simulink library "My_FI_Operations"  (R2023a)
settings: Solver=VariableStepAuto  StartTime=0.0  StopTime=10.0  RelTol=1e-3
settings Model: Creator=kolbe  LastModifiedBy=kolbe
settings DebuggingCC: UnconnectedInputMsg=warning  UnconnectedOutputMsg=warning  UnconnectedLineMsg=warning
settings ModelReferenceCC: EnableRefExpFcnMdlSchedulingChecks=on
settings RTWCC: DLArmComputeVersion=19.05

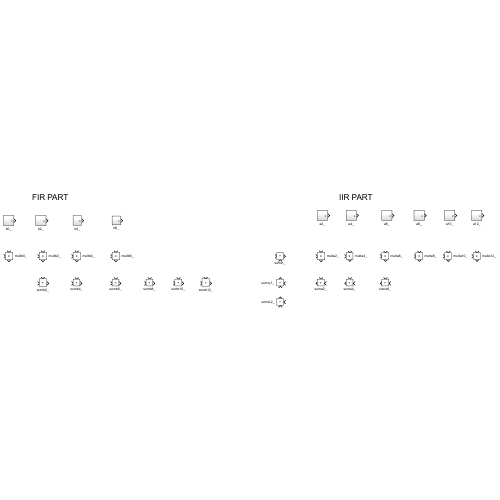
[thumbnail: Simulink's stored preview of the top-level diagram]
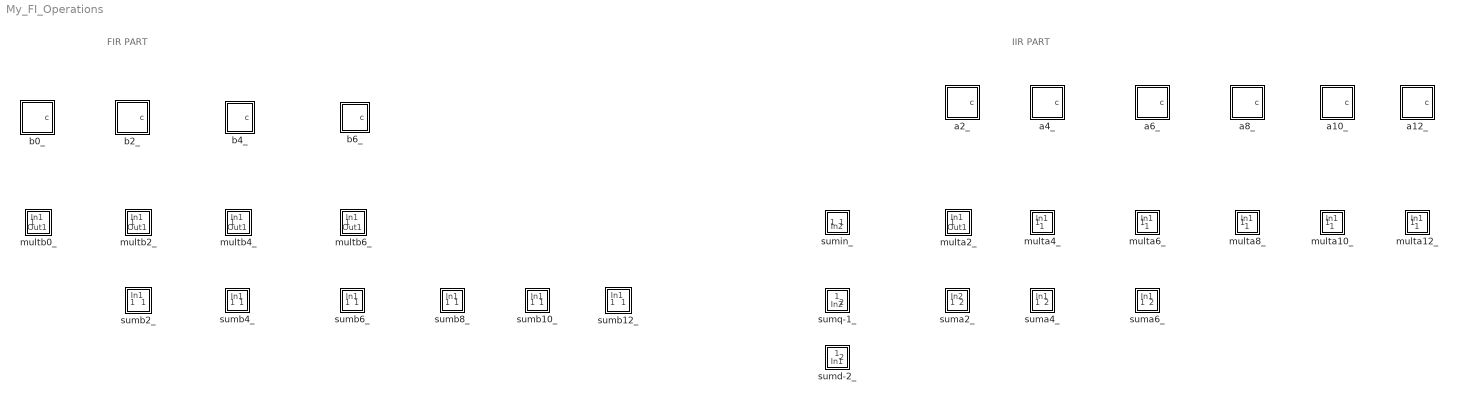
== system My_FI_Operations ==
  note: FIR PART
  note: IIR PART
  a10_ : Subsystem
  a12_ : Subsystem
  a2_ : Subsystem
  a4_ : Subsystem
  a6_ : Subsystem
  a8_ : Subsystem
  b0_ : Subsystem
  b2_ : Subsystem
  b4_ : Subsystem
  b6_ : Subsystem
  multa10_ : Subsystem
      settings: PortSchema="{\"entries\":[{\"content\":{\"sides\":[{\"content\":{\"connectorIds\":[\"In1\"]},\"type\":\"ConnectorPlacement.EquallySpacedRectSide\",\"uuid\":\"423828e0-6700-4575-ac06-a5fb7cb5569f\"},{\"content\":{\"connectorIds\":[],\"side\":\"RIGHT\"},\"type\":\"ConnectorPlacement.EquallySpacedRectSide\",\"uuid\":\"a42db842-eb55-44f2-8f04-0144bc45d908\"},{\"content\":{\"connectorIds\":[\"In2\"],\"side\":\"TOP\"},\"type\":\"ConnectorPlacement.EquallySpacedRectSide\",\"uuid\":\"eef5137d-31f0-46b4-a53b-5aa31464a7f9\"},{\"content\":{\"connectorIds\":[\"Out1\"],\"side\":\"BOTTOM\"},\"type\":\"ConnectorPlacement.EquallySpacedRectSide\",\"uuid\":\"0c804fa9-8d94-49f3-91d8-5fb511150c33\"}]},\"type\":\"ConnectorPlacement.EquallySpacedConnector\",\"uuid\":\"7dd7fe03-b221-4701-a7b2-6552f08320da\"}],\"packageUris\":[\"http://schema.mathworks.com/mf0/Connector/R2020b\"],\"version\":\"1.0\"}"
      mask Display: disp('x')
  multa12_ : Subsystem
      settings: PortSchema="{\"entries\":[{\"content\":{\"sides\":[{\"content\":{\"connectorIds\":[\"In1\"]},\"type\":\"ConnectorPlacement.EquallySpacedRectSide\",\"uuid\":\"423828e0-6700-4575-ac06-a5fb7cb5569f\"},{\"content\":{\"connectorIds\":[],\"side\":\"RIGHT\"},\"type\":\"ConnectorPlacement.EquallySpacedRectSide\",\"uuid\":\"a42db842-eb55-44f2-8f04-0144bc45d908\"},{\"content\":{\"connectorIds\":[\"In2\"],\"side\":\"TOP\"},\"type\":\"ConnectorPlacement.EquallySpacedRectSide\",\"uuid\":\"eef5137d-31f0-46b4-a53b-5aa31464a7f9\"},{\"content\":{\"connectorIds\":[\"Out1\"],\"side\":\"BOTTOM\"},\"type\":\"ConnectorPlacement.EquallySpacedRectSide\",\"uuid\":\"8449918d-02c6-4967-8b4f-9e277713318d\"}]},\"type\":\"ConnectorPlacement.EquallySpacedConnector\",\"uuid\":\"7dd7fe03-b221-4701-a7b2-6552f08320da\"}],\"packageUris\":[\"http://schema.mathworks.com/mf0/Connector/R2020b\"],\"version\":\"1.0\"}"
      mask Display: disp('x')
  multa2_ : Subsystem
      settings: PortSchema="{\"entries\":[{\"content\":{\"sides\":[{\"content\":{\"connectorIds\":[\"In1\"]},\"type\":\"ConnectorPlacement.EquallySpacedRectSide\",\"uuid\":\"423828e0-6700-4575-ac06-a5fb7cb5569f\"},{\"content\":{\"connectorIds\":[],\"side\":\"RIGHT\"},\"type\":\"ConnectorPlacement.EquallySpacedRectSide\",\"uuid\":\"a42db842-eb55-44f2-8f04-0144bc45d908\"},{\"content\":{\"connectorIds\":[\"In2\"],\"side\":\"TOP\"},\"type\":\"ConnectorPlacement.EquallySpacedRectSide\",\"uuid\":\"eef5137d-31f0-46b4-a53b-5aa31464a7f9\"},{\"content\":{\"connectorIds\":[\"Out1\"],\"side\":\"BOTTOM\"},\"type\":\"ConnectorPlacement.EquallySpacedRectSide\",\"uuid\":\"55d96b2a-2b7e-4fdf-a401-8e78f7d2a1aa\"}]},\"type\":\"ConnectorPlacement.EquallySpacedConnector\",\"uuid\":\"7dd7fe03-b221-4701-a7b2-6552f08320da\"}],\"packageUris\":[\"http://schema.mathworks.com/mf0/Connector/R2020b\"],\"version\":\"1.0\"}"
      mask Display: disp('x')
  multa4_ : Subsystem
      settings: PortSchema="{\"entries\":[{\"content\":{\"sides\":[{\"content\":{\"connectorIds\":[\"In1\"]},\"type\":\"ConnectorPlacement.EquallySpacedRectSide\",\"uuid\":\"423828e0-6700-4575-ac06-a5fb7cb5569f\"},{\"content\":{\"connectorIds\":[],\"side\":\"RIGHT\"},\"type\":\"ConnectorPlacement.EquallySpacedRectSide\",\"uuid\":\"a42db842-eb55-44f2-8f04-0144bc45d908\"},{\"content\":{\"connectorIds\":[\"In2\"],\"side\":\"TOP\"},\"type\":\"ConnectorPlacement.EquallySpacedRectSide\",\"uuid\":\"eef5137d-31f0-46b4-a53b-5aa31464a7f9\"},{\"content\":{\"connectorIds\":[\"Out1\"],\"side\":\"BOTTOM\"},\"type\":\"ConnectorPlacement.EquallySpacedRectSide\",\"uuid\":\"24a9476e-4370-431a-bbc5-245c90c7a6e7\"}]},\"type\":\"ConnectorPlacement.EquallySpacedConnector\",\"uuid\":\"7dd7fe03-b221-4701-a7b2-6552f08320da\"}],\"packageUris\":[\"http://schema.mathworks.com/mf0/Connector/R2020b\"],\"version\":\"1.0\"}"
      mask Display: disp('x')
  multa6_ : Subsystem
      settings: PortSchema="{\"entries\":[{\"content\":{\"sides\":[{\"content\":{\"connectorIds\":[\"In1\"]},\"type\":\"ConnectorPlacement.EquallySpacedRectSide\",\"uuid\":\"423828e0-6700-4575-ac06-a5fb7cb5569f\"},{\"content\":{\"connectorIds\":[],\"side\":\"RIGHT\"},\"type\":\"ConnectorPlacement.EquallySpacedRectSide\",\"uuid\":\"a42db842-eb55-44f2-8f04-0144bc45d908\"},{\"content\":{\"connectorIds\":[\"In2\"],\"side\":\"TOP\"},\"type\":\"ConnectorPlacement.EquallySpacedRectSide\",\"uuid\":\"eef5137d-31f0-46b4-a53b-5aa31464a7f9\"},{\"content\":{\"connectorIds\":[\"Out1\"],\"side\":\"BOTTOM\"},\"type\":\"ConnectorPlacement.EquallySpacedRectSide\",\"uuid\":\"47329aef-84bb-47a0-9b32-b12909a392a1\"}]},\"type\":\"ConnectorPlacement.EquallySpacedConnector\",\"uuid\":\"7dd7fe03-b221-4701-a7b2-6552f08320da\"}],\"packageUris\":[\"http://schema.mathworks.com/mf0/Connector/R2020b\"],\"version\":\"1.0\"}"
      mask Display: disp('x')
  multa8_ : Subsystem
      settings: PortSchema="{\"entries\":[{\"content\":{\"sides\":[{\"content\":{\"connectorIds\":[\"In1\"]},\"type\":\"ConnectorPlacement.EquallySpacedRectSide\",\"uuid\":\"423828e0-6700-4575-ac06-a5fb7cb5569f\"},{\"content\":{\"connectorIds\":[],\"side\":\"RIGHT\"},\"type\":\"ConnectorPlacement.EquallySpacedRectSide\",\"uuid\":\"a42db842-eb55-44f2-8f04-0144bc45d908\"},{\"content\":{\"connectorIds\":[\"In2\"],\"side\":\"TOP\"},\"type\":\"ConnectorPlacement.EquallySpacedRectSide\",\"uuid\":\"eef5137d-31f0-46b4-a53b-5aa31464a7f9\"},{\"content\":{\"connectorIds\":[\"Out1\"],\"side\":\"BOTTOM\"},\"type\":\"ConnectorPlacement.EquallySpacedRectSide\",\"uuid\":\"5c073f60-f22f-4cd7-abc5-d0d5f88f0213\"}]},\"type\":\"ConnectorPlacement.EquallySpacedConnector\",\"uuid\":\"7dd7fe03-b221-4701-a7b2-6552f08320da\"}],\"packageUris\":[\"http://schema.mathworks.com/mf0/Connector/R2020b\"],\"version\":\"1.0\"}"
      mask Display: disp('x')
  multb0_ : Subsystem
      settings: PortSchema="{\"entries\":[{\"content\":{\"sides\":[{\"content\":{\"connectorIds\":[\"In1\"]},\"type\":\"ConnectorPlacement.EquallySpacedRectSide\",\"uuid\":\"20461ecc-945a-453b-bec8-f18bcbd4d7ca\"},{\"content\":{\"connectorIds\":[],\"side\":\"RIGHT\"},\"type\":\"ConnectorPlacement.EquallySpacedRectSide\",\"uuid\":\"a806ae65-26a1-4387-823f-a90265b6c751\"},{\"content\":{\"connectorIds\":[\"In2\"],\"side\":\"TOP\"},\"type\":\"ConnectorPlacement.EquallySpacedRectSide\",\"uuid\":\"faa34e1a-fdc6-4b39-b604-acf00955d353\"},{\"content\":{\"connectorIds\":[\"Out1\"],\"side\":\"BOTTOM\"},\"type\":\"ConnectorPlacement.EquallySpacedRectSide\",\"uuid\":\"6d48c7d1-ec45-4610-bf5d-3af7cf103011\"}]},\"type\":\"ConnectorPlacement.EquallySpacedConnector\",\"uuid\":\"f3c21808-e34e-4785-8275-0070ba5b450f\"}],\"packageUris\":[\"http://schema.mathworks.com/mf0/Connector/R2020b\"],\"version\":\"1.0\"}"
      mask Display: disp('x')
  multb2_ : Subsystem
      settings: PortSchema="{\"entries\":[{\"content\":{\"sides\":[{\"content\":{\"connectorIds\":[\"In1\"]},\"type\":\"ConnectorPlacement.EquallySpacedRectSide\",\"uuid\":\"20461ecc-945a-453b-bec8-f18bcbd4d7ca\"},{\"content\":{\"connectorIds\":[],\"side\":\"RIGHT\"},\"type\":\"ConnectorPlacement.EquallySpacedRectSide\",\"uuid\":\"a806ae65-26a1-4387-823f-a90265b6c751\"},{\"content\":{\"connectorIds\":[\"In2\"],\"side\":\"TOP\"},\"type\":\"ConnectorPlacement.EquallySpacedRectSide\",\"uuid\":\"faa34e1a-fdc6-4b39-b604-acf00955d353\"},{\"content\":{\"connectorIds\":[\"Out1\"],\"side\":\"BOTTOM\"},\"type\":\"ConnectorPlacement.EquallySpacedRectSide\",\"uuid\":\"e1b0fef8-c153-494e-8ffe-3515e962a3c5\"}]},\"type\":\"ConnectorPlacement.EquallySpacedConnector\",\"uuid\":\"f3c21808-e34e-4785-8275-0070ba5b450f\"}],\"packageUris\":[\"http://schema.mathworks.com/mf0/Connector/R2020b\"],\"version\":\"1.0\"}"
      mask Display: disp('x')
  multb4_ : Subsystem
      settings: PortSchema="{\"entries\":[{\"content\":{\"sides\":[{\"content\":{\"connectorIds\":[\"In1\"]},\"type\":\"ConnectorPlacement.EquallySpacedRectSide\",\"uuid\":\"20461ecc-945a-453b-bec8-f18bcbd4d7ca\"},{\"content\":{\"connectorIds\":[],\"side\":\"RIGHT\"},\"type\":\"ConnectorPlacement.EquallySpacedRectSide\",\"uuid\":\"a806ae65-26a1-4387-823f-a90265b6c751\"},{\"content\":{\"connectorIds\":[\"In2\"],\"side\":\"TOP\"},\"type\":\"ConnectorPlacement.EquallySpacedRectSide\",\"uuid\":\"faa34e1a-fdc6-4b39-b604-acf00955d353\"},{\"content\":{\"connectorIds\":[\"Out1\"],\"side\":\"BOTTOM\"},\"type\":\"ConnectorPlacement.EquallySpacedRectSide\",\"uuid\":\"234e609c-6b95-41af-91dd-8a06091f2e10\"}]},\"type\":\"ConnectorPlacement.EquallySpacedConnector\",\"uuid\":\"f3c21808-e34e-4785-8275-0070ba5b450f\"}],\"packageUris\":[\"http://schema.mathworks.com/mf0/Connector/R2020b\"],\"version\":\"1.0\"}"
      mask Display: disp('x')
  multb6_ : Subsystem
      settings: PortSchema="{\"entries\":[{\"content\":{\"sides\":[{\"content\":{\"connectorIds\":[\"In1\"]},\"type\":\"ConnectorPlacement.EquallySpacedRectSide\",\"uuid\":\"20461ecc-945a-453b-bec8-f18bcbd4d7ca\"},{\"content\":{\"connectorIds\":[],\"side\":\"RIGHT\"},\"type\":\"ConnectorPlacement.EquallySpacedRectSide\",\"uuid\":\"a806ae65-26a1-4387-823f-a90265b6c751\"},{\"content\":{\"connectorIds\":[\"In2\"],\"side\":\"TOP\"},\"type\":\"ConnectorPlacement.EquallySpacedRectSide\",\"uuid\":\"faa34e1a-fdc6-4b39-b604-acf00955d353\"},{\"content\":{\"connectorIds\":[\"Out1\"],\"side\":\"BOTTOM\"},\"type\":\"ConnectorPlacement.EquallySpacedRectSide\",\"uuid\":\"31f2fa17-ae8c-4166-97ac-b63529612348\"}]},\"type\":\"ConnectorPlacement.EquallySpacedConnector\",\"uuid\":\"f3c21808-e34e-4785-8275-0070ba5b450f\"}],\"packageUris\":[\"http://schema.mathworks.com/mf0/Connector/R2020b\"],\"version\":\"1.0\"}"
      mask Display: disp('x')
  suma2_ : Subsystem
      settings: PortSchema="{\"entries\":[{\"content\":{\"sides\":[{\"content\":{\"connectorIds\":[\"Out1\"]},\"type\":\"ConnectorPlacement.EquallySpacedRectSide\",\"uuid\":\"423828e0-6700-4575-ac06-a5fb7cb5569f\"},{\"content\":{\"connectorIds\":[\"In2\"],\"side\":\"RIGHT\"},\"type\":\"ConnectorPlacement.EquallySpacedRectSide\",\"uuid\":\"a42db842-eb55-44f2-8f04-0144bc45d908\"},{\"content\":{\"connectorIds\":[\"In1\"],\"side\":\"TOP\"},\"type\":\"ConnectorPlacement.EquallySpacedRectSide\",\"uuid\":\"eef5137d-31f0-46b4-a53b-5aa31464a7f9\"}]},\"type\":\"ConnectorPlacement.EquallySpacedConnector\",\"uuid\":\"7dd7fe03-b221-4701-a7b2-6552f08320da\"}],\"packageUris\":[\"http://schema.mathworks.com/mf0/Connector/R2020b\"],\"version\":\"1.0\"}"
      mask Display: disp('+')
  suma4_ : Subsystem
      settings: PortSchema="{\"entries\":[{\"content\":{\"sides\":[{\"content\":{\"connectorIds\":[\"Out1\"]},\"type\":\"ConnectorPlacement.EquallySpacedRectSide\",\"uuid\":\"423828e0-6700-4575-ac06-a5fb7cb5569f\"},{\"content\":{\"connectorIds\":[\"In2\"],\"side\":\"RIGHT\"},\"type\":\"ConnectorPlacement.EquallySpacedRectSide\",\"uuid\":\"a42db842-eb55-44f2-8f04-0144bc45d908\"},{\"content\":{\"connectorIds\":[\"In1\"],\"side\":\"TOP\"},\"type\":\"ConnectorPlacement.EquallySpacedRectSide\",\"uuid\":\"eef5137d-31f0-46b4-a53b-5aa31464a7f9\"}]},\"type\":\"ConnectorPlacement.EquallySpacedConnector\",\"uuid\":\"7dd7fe03-b221-4701-a7b2-6552f08320da\"}],\"packageUris\":[\"http://schema.mathworks.com/mf0/Connector/R2020b\"],\"version\":\"1.0\"}"
      mask Display: disp('+')
  suma6_ : Subsystem
      settings: PortSchema="{\"entries\":[{\"content\":{\"sides\":[{\"content\":{\"connectorIds\":[\"Out1\"]},\"type\":\"ConnectorPlacement.EquallySpacedRectSide\",\"uuid\":\"423828e0-6700-4575-ac06-a5fb7cb5569f\"},{\"content\":{\"connectorIds\":[\"In2\"],\"side\":\"RIGHT\"},\"type\":\"ConnectorPlacement.EquallySpacedRectSide\",\"uuid\":\"a42db842-eb55-44f2-8f04-0144bc45d908\"},{\"content\":{\"connectorIds\":[\"In1\"],\"side\":\"TOP\"},\"type\":\"ConnectorPlacement.EquallySpacedRectSide\",\"uuid\":\"eef5137d-31f0-46b4-a53b-5aa31464a7f9\"}]},\"type\":\"ConnectorPlacement.EquallySpacedConnector\",\"uuid\":\"7dd7fe03-b221-4701-a7b2-6552f08320da\"}],\"packageUris\":[\"http://schema.mathworks.com/mf0/Connector/R2020b\"],\"version\":\"1.0\"}"
      mask Display: disp('+')
  sumb10_ : Subsystem
      settings: PortSchema="{\"entries\":[{\"content\":{\"sides\":[{\"content\":{\"connectorIds\":[\"In1\"]},\"type\":\"ConnectorPlacement.EquallySpacedRectSide\",\"uuid\":\"20461ecc-945a-453b-bec8-f18bcbd4d7ca\"},{\"content\":{\"connectorIds\":[\"Out1\"],\"side\":\"RIGHT\"},\"type\":\"ConnectorPlacement.EquallySpacedRectSide\",\"uuid\":\"a806ae65-26a1-4387-823f-a90265b6c751\"},{\"content\":{\"connectorIds\":[\"In2\"],\"side\":\"TOP\"},\"type\":\"ConnectorPlacement.EquallySpacedRectSide\",\"uuid\":\"faa34e1a-fdc6-4b39-b604-acf00955d353\"}]},\"type\":\"ConnectorPlacement.EquallySpacedConnector\",\"uuid\":\"f3c21808-e34e-4785-8275-0070ba5b450f\"}],\"packageUris\":[\"http://schema.mathworks.com/mf0/Connector/R2020b\"],\"version\":\"1.0\"}"
      mask Display: disp('+')
  sumb12_ : Subsystem
      settings: PortSchema="{\"entries\":[{\"content\":{\"sides\":[{\"content\":{\"connectorIds\":[\"In1\"]},\"type\":\"ConnectorPlacement.EquallySpacedRectSide\",\"uuid\":\"20461ecc-945a-453b-bec8-f18bcbd4d7ca\"},{\"content\":{\"connectorIds\":[\"Out1\"],\"side\":\"RIGHT\"},\"type\":\"ConnectorPlacement.EquallySpacedRectSide\",\"uuid\":\"a806ae65-26a1-4387-823f-a90265b6c751\"},{\"content\":{\"connectorIds\":[\"In2\"],\"side\":\"TOP\"},\"type\":\"ConnectorPlacement.EquallySpacedRectSide\",\"uuid\":\"faa34e1a-fdc6-4b39-b604-acf00955d353\"}]},\"type\":\"ConnectorPlacement.EquallySpacedConnector\",\"uuid\":\"f3c21808-e34e-4785-8275-0070ba5b450f\"}],\"packageUris\":[\"http://schema.mathworks.com/mf0/Connector/R2020b\"],\"version\":\"1.0\"}"
      mask Display: disp('+')
  sumb2_ : Subsystem
      settings: PortSchema="{\"entries\":[{\"content\":{\"sides\":[{\"content\":{\"connectorIds\":[\"In1\"]},\"type\":\"ConnectorPlacement.EquallySpacedRectSide\",\"uuid\":\"20461ecc-945a-453b-bec8-f18bcbd4d7ca\"},{\"content\":{\"connectorIds\":[\"Out1\"],\"side\":\"RIGHT\"},\"type\":\"ConnectorPlacement.EquallySpacedRectSide\",\"uuid\":\"a806ae65-26a1-4387-823f-a90265b6c751\"},{\"content\":{\"connectorIds\":[\"In2\"],\"side\":\"TOP\"},\"type\":\"ConnectorPlacement.EquallySpacedRectSide\",\"uuid\":\"faa34e1a-fdc6-4b39-b604-acf00955d353\"}]},\"type\":\"ConnectorPlacement.EquallySpacedConnector\",\"uuid\":\"f3c21808-e34e-4785-8275-0070ba5b450f\"}],\"packageUris\":[\"http://schema.mathworks.com/mf0/Connector/R2020b\"],\"version\":\"1.0\"}"
      mask Display: disp('+')
  sumb4_ : Subsystem
      settings: PortSchema="{\"entries\":[{\"content\":{\"sides\":[{\"content\":{\"connectorIds\":[\"In1\"]},\"type\":\"ConnectorPlacement.EquallySpacedRectSide\",\"uuid\":\"20461ecc-945a-453b-bec8-f18bcbd4d7ca\"},{\"content\":{\"connectorIds\":[\"Out1\"],\"side\":\"RIGHT\"},\"type\":\"ConnectorPlacement.EquallySpacedRectSide\",\"uuid\":\"a806ae65-26a1-4387-823f-a90265b6c751\"},{\"content\":{\"connectorIds\":[\"In2\"],\"side\":\"TOP\"},\"type\":\"ConnectorPlacement.EquallySpacedRectSide\",\"uuid\":\"faa34e1a-fdc6-4b39-b604-acf00955d353\"}]},\"type\":\"ConnectorPlacement.EquallySpacedConnector\",\"uuid\":\"f3c21808-e34e-4785-8275-0070ba5b450f\"}],\"packageUris\":[\"http://schema.mathworks.com/mf0/Connector/R2020b\"],\"version\":\"1.0\"}"
      mask Display: disp('+')
  sumb6_ : Subsystem
      settings: PortSchema="{\"entries\":[{\"content\":{\"sides\":[{\"content\":{\"connectorIds\":[\"In1\"]},\"type\":\"ConnectorPlacement.EquallySpacedRectSide\",\"uuid\":\"20461ecc-945a-453b-bec8-f18bcbd4d7ca\"},{\"content\":{\"connectorIds\":[\"Out1\"],\"side\":\"RIGHT\"},\"type\":\"ConnectorPlacement.EquallySpacedRectSide\",\"uuid\":\"a806ae65-26a1-4387-823f-a90265b6c751\"},{\"content\":{\"connectorIds\":[\"In2\"],\"side\":\"TOP\"},\"type\":\"ConnectorPlacement.EquallySpacedRectSide\",\"uuid\":\"faa34e1a-fdc6-4b39-b604-acf00955d353\"}]},\"type\":\"ConnectorPlacement.EquallySpacedConnector\",\"uuid\":\"f3c21808-e34e-4785-8275-0070ba5b450f\"}],\"packageUris\":[\"http://schema.mathworks.com/mf0/Connector/R2020b\"],\"version\":\"1.0\"}"
      mask Display: disp('+')
  sumb8_ : Subsystem
      settings: PortSchema="{\"entries\":[{\"content\":{\"sides\":[{\"content\":{\"connectorIds\":[\"In1\"]},\"type\":\"ConnectorPlacement.EquallySpacedRectSide\",\"uuid\":\"20461ecc-945a-453b-bec8-f18bcbd4d7ca\"},{\"content\":{\"connectorIds\":[\"Out1\"],\"side\":\"RIGHT\"},\"type\":\"ConnectorPlacement.EquallySpacedRectSide\",\"uuid\":\"a806ae65-26a1-4387-823f-a90265b6c751\"},{\"content\":{\"connectorIds\":[\"In2\"],\"side\":\"TOP\"},\"type\":\"ConnectorPlacement.EquallySpacedRectSide\",\"uuid\":\"faa34e1a-fdc6-4b39-b604-acf00955d353\"}]},\"type\":\"ConnectorPlacement.EquallySpacedConnector\",\"uuid\":\"f3c21808-e34e-4785-8275-0070ba5b450f\"}],\"packageUris\":[\"http://schema.mathworks.com/mf0/Connector/R2020b\"],\"version\":\"1.0\"}"
      mask Display: disp('+')
  sumd-2_ : Subsystem
      settings: PortSchema="{\"entries\":[{\"content\":{\"sides\":[{\"content\":{\"connectorIds\":[]},\"type\":\"ConnectorPlacement.EquallySpacedRectSide\",\"uuid\":\"423828e0-6700-4575-ac06-a5fb7cb5569f\"},{\"content\":{\"connectorIds\":[\"In2\"],\"side\":\"RIGHT\"},\"type\":\"ConnectorPlacement.EquallySpacedRectSide\",\"uuid\":\"a42db842-eb55-44f2-8f04-0144bc45d908\"},{\"content\":{\"connectorIds\":[\"Out1\"],\"side\":\"TOP\"},\"type\":\"ConnectorPlacement.EquallySpacedRectSide\",\"uuid\":\"eef5137d-31f0-46b4-a53b-5aa31464a7f9\"},{\"content\":{\"connectorIds\":[\"In1\"],\"side\":\"BOTTOM\"},\"type\":\"ConnectorPlacement.EquallySpacedRectSide\",\"uuid\":\"0a29e77a-4bdf-45d0-8a25-1103c3446174\"}]},\"type\":\"ConnectorPlacement.EquallySpacedConnector\",\"uuid\":\"7dd7fe03-b221-4701-a7b2-6552f08320da\"}],\"packageUris\":[\"http://schema.mathworks.com/mf0/Connector/R2020b\"],\"version\":\"1.0\"}"
      mask Display: disp('+')
  sumin_ : Subsystem
      settings: PortSchema="{\"entries\":[{\"content\":{\"sides\":[{\"content\":{\"connectorIds\":[\"In1\"]},\"type\":\"ConnectorPlacement.EquallySpacedRectSide\",\"uuid\":\"423828e0-6700-4575-ac06-a5fb7cb5569f\"},{\"content\":{\"connectorIds\":[\"Out1\"],\"side\":\"RIGHT\"},\"type\":\"ConnectorPlacement.EquallySpacedRectSide\",\"uuid\":\"a42db842-eb55-44f2-8f04-0144bc45d908\"},{\"content\":{\"connectorIds\":[],\"side\":\"TOP\"},\"type\":\"ConnectorPlacement.EquallySpacedRectSide\",\"uuid\":\"eef5137d-31f0-46b4-a53b-5aa31464a7f9\"},{\"content\":{\"connectorIds\":[\"In2\"],\"side\":\"BOTTOM\"},\"type\":\"ConnectorPlacement.EquallySpacedRectSide\",\"uuid\":\"f3760898-0e2b-4385-8757-2cc61988fa54\"}]},\"type\":\"ConnectorPlacement.EquallySpacedConnector\",\"uuid\":\"7dd7fe03-b221-4701-a7b2-6552f08320da\"}],\"packageUris\":[\"http://schema.mathworks.com/mf0/Connector/R2020b\"],\"version\":\"1.0\"}"
      mask Display: disp('+')
  sumq-1_ : Subsystem
      settings: PortSchema="{\"entries\":[{\"content\":{\"sides\":[{\"content\":{\"connectorIds\":[]},\"type\":\"ConnectorPlacement.EquallySpacedRectSide\",\"uuid\":\"423828e0-6700-4575-ac06-a5fb7cb5569f\"},{\"content\":{\"connectorIds\":[\"In2\"],\"side\":\"RIGHT\"},\"type\":\"ConnectorPlacement.EquallySpacedRectSide\",\"uuid\":\"a42db842-eb55-44f2-8f04-0144bc45d908\"},{\"content\":{\"connectorIds\":[\"Out1\"],\"side\":\"TOP\"},\"type\":\"ConnectorPlacement.EquallySpacedRectSide\",\"uuid\":\"eef5137d-31f0-46b4-a53b-5aa31464a7f9\"},{\"content\":{\"connectorIds\":[\"In1\"],\"side\":\"BOTTOM\"},\"type\":\"ConnectorPlacement.EquallySpacedRectSide\",\"uuid\":\"2873f229-5340-47da-9b40-109923f96826\"}]},\"type\":\"ConnectorPlacement.EquallySpacedConnector\",\"uuid\":\"7dd7fe03-b221-4701-a7b2-6552f08320da\"}],\"packageUris\":[\"http://schema.mathworks.com/mf0/Connector/R2020b\"],\"version\":\"1.0\"}"
      mask Display: disp('+')

== system My_FI_Operations/a10_ ==
  a10_ : Constant  Value=-1.218261718750000  OutDataTypeStr=fixdt(1,15,11)
  c : Outport
  wires:
  a10_/1 -> c/1

== system My_FI_Operations/a12_ ==
  a12_ : Constant  Value=-0.203125000000000  OutDataTypeStr=fixdt(1,15,11)
  c : Outport
  wires:
  a12_/1 -> c/1

== system My_FI_Operations/a2_ ==
  a2_ : Constant  Value=-3.291503906250000  OutDataTypeStr=fixdt(1,15,11)
  c : Outport
  wires:
  a2_/1 -> c/1

== system My_FI_Operations/a4_ ==
  a4_ : Constant  Value=-5.456054687500000  OutDataTypeStr=fixdt(1,15,11)
  c : Outport
  wires:
  a4_/1 -> c/1

== system My_FI_Operations/a6_ ==
  a6_ : Constant  Value=-5.414062500000000  OutDataTypeStr=fixdt(1,15,11)
  c : Outport
  wires:
  a6_/1 -> c/1

== system My_FI_Operations/a8_ ==
  a8_ : Constant  Value=-3.354492187500000  OutDataTypeStr=fixdt(1,15,11)
  c : Outport
  wires:
  a8_/1 -> c/1

== system My_FI_Operations/b0_ ==
  b0_ : Constant  Value=0.004394531250000  OutDataTypeStr=fixdt(1,12,11)
  c : Outport
  wires:
  b0_/1 -> c/1

== system My_FI_Operations/b2_ ==
  b2_ : Constant  Value=-0.010742187500000  OutDataTypeStr=fixdt(1,12,11)
  c : Outport
  wires:
  b2_/1 -> c/1

== system My_FI_Operations/b4_ ==
  b4_ : Constant  Value=0.018554687500000  OutDataTypeStr=fixdt(1,12,11)
  c : Outport
  wires:
  b4_/1 -> c/1

== system My_FI_Operations/b6_ ==
  b6_ : Constant  Value=-0.021484375000000  OutDataTypeStr=fixdt(1,12,11)
  c : Outport
  wires:
  b6_/1 -> c/1

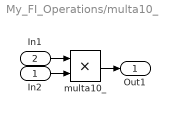
== system My_FI_Operations/multa10_ ==
  In2 : Inport
  In1 : Inport  Port=2
  multa10_ : Product  OutDataTypeStr=fixdt(1,26,24-10+FL)  RndMeth=Nearest  SaturateOnIntegerOverflow=on
  Out1 : Outport
  wires:
  In1/1 -> multa10_/1
  In2/1 -> multa10_/2
  multa10_/1 -> Out1/1

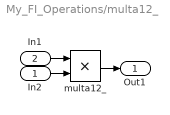
== system My_FI_Operations/multa12_ ==
  In2 : Inport
  In1 : Inport  Port=2
  multa12_ : Product  OutDataTypeStr=fixdt(1,27,26-10+FL)  RndMeth=Nearest  SaturateOnIntegerOverflow=on
  Out1 : Outport
  wires:
  In2/1 -> multa12_/2
  In1/1 -> multa12_/1
  multa12_/1 -> Out1/1

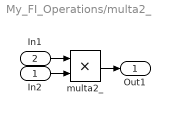
== system My_FI_Operations/multa2_ ==
  In2 : Inport
  In1 : Inport  Port=2
  multa2_ : Product  OutDataTypeStr=fixdt(1,39,36-10+FL)  RndMeth=Nearest  SaturateOnIntegerOverflow=on
  Out1 : Outport
  wires:
  In2/1 -> multa2_/2
  In1/1 -> multa2_/1
  multa2_/1 -> Out1/1

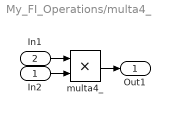
== system My_FI_Operations/multa4_ ==
  In2 : Inport
  In1 : Inport  Port=2
  multa4_ : Product  OutDataTypeStr=fixdt(1,44,40-10+FL)  RndMeth=Nearest  SaturateOnIntegerOverflow=on
  Out1 : Outport
  wires:
  In1/1 -> multa4_/1
  multa4_/1 -> Out1/1
  In2/1 -> multa4_/2

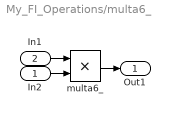
== system My_FI_Operations/multa6_ ==
  In2 : Inport
  In1 : Inport  Port=2
  multa6_ : Product  OutDataTypeStr=fixdt(1,29,25-10+FL)  RndMeth=Nearest  SaturateOnIntegerOverflow=on
  Out1 : Outport
  wires:
  In1/1 -> multa6_/1
  In2/1 -> multa6_/2
  multa6_/1 -> Out1/1

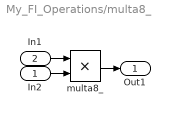
== system My_FI_Operations/multa8_ ==
  In2 : Inport
  In1 : Inport  Port=2
  multa8_ : Product  OutDataTypeStr=fixdt(1,36,33-10+FL)  RndMeth=Nearest  SaturateOnIntegerOverflow=on
  Out1 : Outport
  wires:
  In1/1 -> multa8_/1
  In2/1 -> multa8_/2
  multa8_/1 -> Out1/1

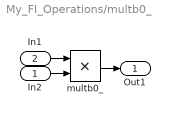
== system My_FI_Operations/multb0_ ==
  In2 : Inport
  In1 : Inport  Port=2
  multb0_ : Product  OutDataTypeStr=fixdt(1,22,21-10+FL)  RndMeth=Nearest  SaturateOnIntegerOverflow=on
  Out1 : Outport
  wires:
  In1/1 -> multb0_/1
  multb0_/1 -> Out1/1
  In2/1 -> multb0_/2

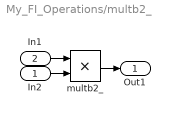
== system My_FI_Operations/multb2_ ==
  In2 : Inport
  In1 : Inport  Port=2
  multb2_ : Product  OutDataTypeStr=fixdt(1,21,20-10+FL)  RndMeth=Nearest  SaturateOnIntegerOverflow=on
  Out1 : Outport
  wires:
  multb2_/1 -> Out1/1
  In2/1 -> multb2_/2
  In1/1 -> multb2_/1

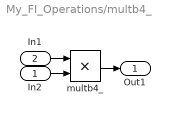
== system My_FI_Operations/multb4_ ==
  In2 : Inport
  In1 : Inport  Port=2
  multb4_ : Product  OutDataTypeStr=fixdt(1,21,20-10+FL)  RndMeth=Nearest  SaturateOnIntegerOverflow=on
  Out1 : Outport
  wires:
  multb4_/1 -> Out1/1
  In1/1 -> multb4_/1
  In2/1 -> multb4_/2

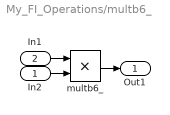
== system My_FI_Operations/multb6_ ==
  In2 : Inport
  In1 : Inport  Port=2
  multb6_ : Product  OutDataTypeStr=fixdt(1,20,19-10+FL)  RndMeth=Nearest  SaturateOnIntegerOverflow=on
  Out1 : Outport
  wires:
  In1/1 -> multb6_/1
  multb6_/1 -> Out1/1
  In2/1 -> multb6_/2

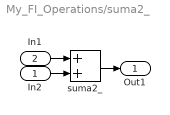
== system My_FI_Operations/suma2_ ==
  In2 : Inport
  In1 : Inport  Port=2
  suma2_ : Sum  OutDataTypeStr=fixdt(1,33,29-10+FL)  RndMeth=Nearest  SaturateOnIntegerOverflow=on
  Out1 : Outport
  wires:
  In2/1 -> suma2_/2
  suma2_/1 -> Out1/1
  In1/1 -> suma2_/1

== system My_FI_Operations/suma4_ ==
  In1 : Inport
  In2 : Inport  Port=2
  suma4_ : Sum  OutDataTypeStr=fixdt(1,42,38-10+FL)  RndMeth=Nearest  SaturateOnIntegerOverflow=on
  Out1 : Outport
  wires:
  suma4_/1 -> Out1/1
  In2/1 -> suma4_/2
  In1/1 -> suma4_/1

== system My_FI_Operations/suma6_ ==
  In1 : Inport
  In2 : Inport  Port=2
  suma6_ : Sum  OutDataTypeStr=fixdt(1,28,24-10+FL)  RndMeth=Nearest  SaturateOnIntegerOverflow=on
  Out1 : Outport
  wires:
  In1/1 -> suma6_/1
  In2/1 -> suma6_/2
  suma6_/1 -> Out1/1

== system My_FI_Operations/sumb10_ ==
  In2 : Inport
  In1 : Inport  Port=2
  sumb10_ : Sum  OutDataTypeStr=fixdt(1,22,21-10+FL)  RndMeth=Nearest  SaturateOnIntegerOverflow=on
  Out1 : Outport
  wires:
  In1/1 -> sumb10_/1
  In2/1 -> sumb10_/2
  sumb10_/1 -> Out1/1

== system My_FI_Operations/sumb12_ ==
  In2 : Inport
  In1 : Inport  Port=2
  sumb12_ : Sum  OutDataTypeStr=fixdt(1,22,21-10+FL)  RndMeth=Nearest  SaturateOnIntegerOverflow=on
  Out1 : Outport
  wires:
  In1/1 -> sumb12_/1
  sumb12_/1 -> Out1/1
  In2/1 -> sumb12_/2

== system My_FI_Operations/sumb2_ ==
  In2 : Inport
  In1 : Inport  Port=2
  sumb2_ : Sum  OutDataTypeStr=fixdt(1,22,21-10+FL)  RndMeth=Nearest  SaturateOnIntegerOverflow=on
  Out1 : Outport
  wires:
  In1/1 -> sumb2_/1
  In2/1 -> sumb2_/2
  sumb2_/1 -> Out1/1

== system My_FI_Operations/sumb4_ ==
  In2 : Inport
  In1 : Inport  Port=2
  sumb4_ : Sum  OutDataTypeStr=fixdt(1,22,21-10+FL)  RndMeth=Nearest  SaturateOnIntegerOverflow=on
  Out1 : Outport
  wires:
  In1/1 -> sumb4_/1
  In2/1 -> sumb4_/2
  sumb4_/1 -> Out1/1

== system My_FI_Operations/sumb6_ ==
  In2 : Inport
  In1 : Inport  Port=2
  sumb6_ : Sum  OutDataTypeStr=fixdt(1,22,21-10+FL)  RndMeth=Nearest  SaturateOnIntegerOverflow=on
  Out1 : Outport
  wires:
  sumb6_/1 -> Out1/1
  In1/1 -> sumb6_/1
  In2/1 -> sumb6_/2

== system My_FI_Operations/sumb8_ ==
  In2 : Inport
  In1 : Inport  Port=2
  sumb8_ : Sum  OutDataTypeStr=fixdt(1,22,21-10+FL)  RndMeth=Nearest  SaturateOnIntegerOverflow=on
  Out1 : Outport
  wires:
  sumb8_/1 -> Out1/1
  In1/1 -> sumb8_/1
  In2/1 -> sumb8_/2

== system My_FI_Operations/sumd-2_ ==
  In1 : Inport
  In2 : Inport  Port=2
  sumd-2_ : Sum  OutDataTypeStr=fixdt(1,34,30-10+FL)  RndMeth=Nearest
  Out1 : Outport
  wires:
  In2/1 -> sumd-2_/2
  sumd-2_/1 -> Out1/1
  In1/1 -> sumd-2_/1

== system My_FI_Operations/sumin_ ==
  In1 : Inport
  In2 : Inport  Port=2
  sumin_ : Sum  OutDataTypeStr=fixdt(1,36,34-10+FL)  RndMeth=Nearest  SaturateOnIntegerOverflow=on
  Out1 : Outport
  wires:
  In2/1 -> sumin_/2
  In1/1 -> sumin_/1
  sumin_/1 -> Out1/1

== system My_FI_Operations/sumq-1_ ==
  In2 : Inport
  In1 : Inport  Port=2
  sumq-1_ : Sum  OutDataTypeStr=fixdt(1,39,35-10+FL)  RndMeth=Nearest  SaturateOnIntegerOverflow=on
  Out1 : Outport
  wires:
  sumq-1_/1 -> Out1/1
  In2/1 -> sumq-1_/2
  In1/1 -> sumq-1_/1
